simulink model "PMfinal"  (R2018a)
settings: Solver=VariableStepDiscrete  StartTime=0.0  StopTime=10.0  RelTol=1e-3
libraries: powerlib x16, simulink x3, powerlib_meascontrol x1
settings Model: Creator=enes_  LastModifiedBy=enes_

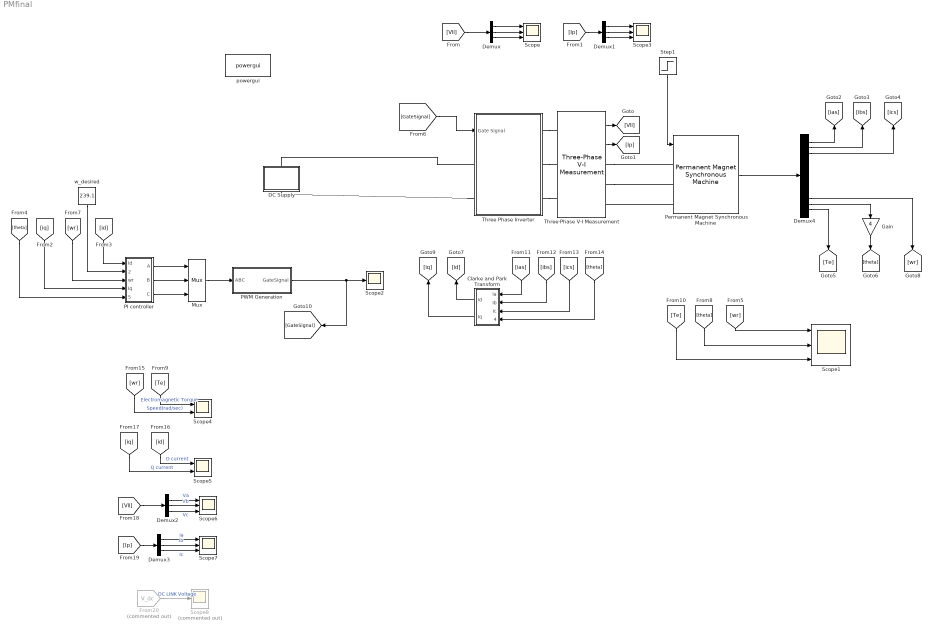
== system PMfinal ==
  Clarke and Park Transform : Subsystem
  DC Supply : Subsystem
  Demux{,1..3} (4 alike) : Demux  Outputs=3
  Demux4 : Demux  Outputs=13
  From20 : From  Commented=on  GotoTag=V_dc  TagVisibility=global
  Gain : Gain  Gain=4
  Mux : Mux  Inputs=3
  PI controller : Subsystem
  PWM Generation : Subsystem
  Permanent Magnet Synchronous Machine : powerlib/Machines/Permanent Magnet Synchronous Machine  NbPhases=3  FluxDistribution=Sinusoidal  RotorType=Round  MechanicalLoad=Torque Tm  PresetModel=No  ShowDetailedParameters=on  MeasurementBus=off  Resistance=50e-3  Inductance=8.5e-3  dqInductances=[500e-6,500e-6]  La=500e-6  MachineConstant=Flux linkage established by magnets (V.s)  Flux=0.2  VoltageCst=145.1039  TorqueCst=1.2  Flat=120  Mechanical=[10 0 4 0]  PolePairs=4  InitialConditions=[266,0, 0,0]  InitialConditions5ph=[266 0 0 0 0 0]  TsPowergui=0  TsBlock=-1  RefAngle=Aligned with phase A axis (original Park)
  Scope{,1,3,6..7} (5 alike) : Scope  NumInputPorts=3
  Scope2 : Scope
  Scope4 : Scope  NumInputPorts=2
  Scope5 : Scope  NumInputPorts=2
  Scope8 : Scope  Commented=on
  Step1 : Step  Time=.1  After=60  SampleTime=1e-6
  Three Phase Inverter : Subsystem  RequirementInfo="{}  %GIDa_97822f1e_2a67_44f0_8b0b_8fc93499e893"
  Three-Phase V-I Measurement : powerlib/Measurements/Three-Phase V-I Measurement  VoltageMeasurement=phase-to-phase  SetLabelV=off  LabelV=Vabc  Vpu=off  VpuLL=off  CurrentMeasurement=yes  SetLabelI=off  LabelI=Iabc  Ipu=off  Pbase=100e6  Vbase=500e3  OutputType=Complex  PhasorSimulation=off  PSBequivalent=0
      settings: SourceProductName=Simscape Electrical
  powergui : powerlib/powergui  Priority=1  SimulationMode=Discrete  SampleTime=1e-6  frequency=60  Iterations=50  frequencyindice=0  Pbase=100e6  ErrMax=1e-4  UnitsV=kV  UnitsW=MW  buscounter=0  FunctionMessages=off  echomessages=off  EnableUseOfTLC=off  CurrentSourceSwitches=off  DisableSnubberDevices=off  DisableRonSwitches=off  DisableVfSwitches=off  DisplayEquations=off  SolverType=Tustin/Backward Euler (TBE)  Interpol=off  ExternalGateDelay=off  methode=off  Ts=100  x0status=blocks  SPID=on  SwTol=0  HookPort=off  RestoreLinks=warning  ResistiveCurrentMeasurement=off  Frange=[0:2:500]  Ylog=off  Xlog=on  ShowGrid=off  save=off  variable=ZData  structure=0  ZoomFFT=off  StartTime=0.0  cycles=1  DisplayStyle=1  fundamental=60  FreqAxis=off  MaxFrequency=1000  frequencyindicesteady=1  RmsSteady=1  display=off
  w_desired : Constant  Value=239.1
  wires:
  Step1/1 -> Permanent Magnet Synchronous Machine/1
  Three-Phase V-I Measurement/1 -> [Vll]
  [Vll] -> Demux/1
  Demux/1 -> Scope/1
  Demux/2 -> Scope/2
  Demux/3 -> Scope/3
  Three-Phase V-I Measurement/2 -> [Ip]
  [Ip] -> Demux1/1
  Demux1/1 -> Scope3/1
  Demux1/2 -> Scope3/2
  Demux1/3 -> Scope3/3
  Permanent Magnet Synchronous Machine/1 -> Demux4/1
  Demux4/1 -> [ias]
  Demux4/2 -> [ibs]
  Demux4/3 -> [ics]
  Demux4/13 -> [Te]
  Demux4/12 -> Gain/1
  Demux4/11 -> [wr]
  Gain/1 -> [theta]
  [wr] -> Scope1/1
  [theta] -> Scope1/2
  [Te] -> Scope1/3
  PWM Generation/1("GateSignal ") -> Scope2/1, [GateSignal]
  Mux/1 -> PWM Generation/1(ABC)
  [GateSignal] -> Three Phase Inverter/1(Gate Signal)
  [ias] -> Clarke and Park Transform/1(Ia)
  [ibs] -> Clarke and Park Transform/2(Ib)
  [ics] -> Clarke and Park Transform/3(Ic)
  [theta] -> Clarke and Park Transform/4(Theta)
  Clarke and Park Transform/1(Id) -> [id]
  Clarke and Park Transform/2(Iq) -> [iq]
  [id] -> PI controller/1(Id)
  w_desired/1 -> PI controller/2(w_ref)
  [wr] -> PI controller/3(wr)
  [iq] -> PI controller/4(Iq)
  [theta] -> PI controller/5(Theta)
  PI controller/1(A) -> Mux/1
  PI controller/2(B) -> Mux/2
  PI controller/3(C) -> Mux/3
  [Te] -> Scope4/1  "Electromagnetic Torque"
  [wr] -> Scope4/2  "Speed(rad/sec)"
  [id] -> Scope5/1  "D current"
  [iq] -> Scope5/2  "Q current"
  Demux3/2 -> Scope7/2  "Ib"
  Demux2/2 -> Scope6/2  "Vb"
  [Vll] -> Demux2/1
  Demux3/1 -> Scope7/1  "Ia"
  Demux2/3 -> Scope6/3  "Vc"
  [Ip] -> Demux3/1
  Demux3/3 -> Scope7/3  "Ic"
  Demux2/1 -> Scope6/1  "Va"
  From20/1 -> Scope8/1  "DC LINK Voltage"
  connections:
  Three Phase Inverter/LConn2 -- DC Supply/LConn1
  DC Supply/RConn1 -- Three Phase Inverter/LConn1
  Three-Phase V-I Measurement/RConn1 -- Permanent Magnet Synchronous Machine/LConn1
  Three-Phase V-I Measurement/RConn2 -- Permanent Magnet Synchronous Machine/LConn2
  Permanent Magnet Synchronous Machine/LConn3 -- Three-Phase V-I Measurement/RConn3
  Three Phase Inverter/RConn1 -- Three-Phase V-I Measurement/LConn1
  Three Phase Inverter/RConn2 -- Three-Phase V-I Measurement/LConn2
  Three Phase Inverter/RConn3 -- Three-Phase V-I Measurement/LConn3

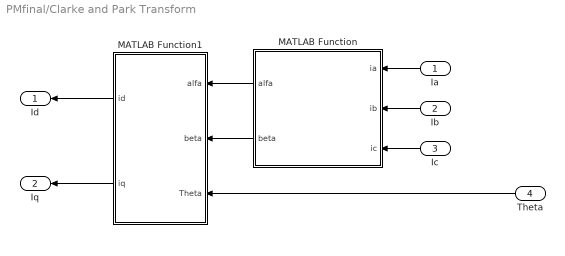
== system PMfinal/Clarke and Park Transform ==
  Ia : Inport
  Ib : Inport  Port=2
  Ic : Inport  Port=3
  Theta : Inport  Port=4
  MATLAB Function : MATLAB Function  TreatAsAtomicUnit=on
  MATLAB Function1 : MATLAB Function  TreatAsAtomicUnit=on
  Id : Outport
  Iq : Outport  Port=2
  wires:
  Ib/1 -> MATLAB Function/2(ib)
  MATLAB Function/2(beta) -> MATLAB Function1/2(beta)
  Ia/1 -> MATLAB Function/1(ia)
  MATLAB Function/1(alfa) -> MATLAB Function1/1(alfa)
  Theta/1 -> MATLAB Function1/3(Theta)
  MATLAB Function1/2(iq) -> Iq/1
  Ic/1 -> MATLAB Function/3(ic)
  MATLAB Function1/1(id) -> Id/1

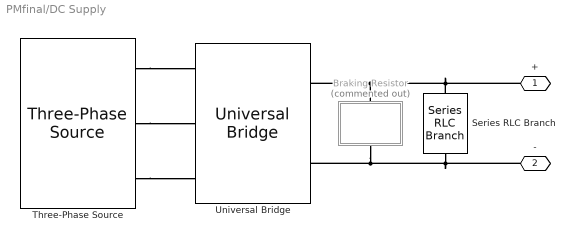
== system PMfinal/DC Supply ==
  "Braking Resistor " : Subsystem  Commented=on
  Series RLC Branch : powerlib/Elements/Series RLC Branch  LConnTagsString=__new0  RConnTagsString=__new0  BranchType=C  Resistance=1  Inductance=1e-3  SetiL0=off  InitialCurrent=0  Capacitance=330e-3  Setx0=off  InitialVoltage=0  Measurements=None
      settings: SourceProductName=Simscape Electrical
  "Three-Phase Source " : powerlib/Electrical Sources/Three-Phase Source  InternalConnection=Yg  VoltagePhases=off  Voltage=400  PhaseAngle=0  Voltage_phases=[25e3 25e3 25e3]/sqrt(3)  PhaseAngles_phases=[0 -120 +120]  Frequency=50  NonIdealSource=off  SpecifyImpedance=off  Resistance=0  Inductance=0  ShortCircuitLevel=100e6  BaseVoltage=25e3  XRratio=7  BusType=swing  Pref=10e3  Qref=0  Prefabc=[10e3, 10e3, 10e3]  Qrefabc=[0, 0, 0]  Qmin=-inf  Qmax=inf
      settings: SourceProductName=Simscape Electrical
  "Universal Bridge " : powerlib/Power Electronics/Universal Bridge  Arms=3  SnubberResistance=1e5  SnubberCapacitance=inf  Device=Diodes  Ron=1e-3  Lon=0  ForwardVoltages="[  0  0  ]"  ForwardVoltage=0  GTOparameters=[ 10e-6 , 20e-6 ]  IGBTparameters=[ 1e-6 , 2e-6 ]  Measurements=All voltages and currents  Measurements_2=None  converterType=Rectifier
      settings: SourceProductName=Simscape Electrical
  + : PMIOPort  Side=Right
  - : PMIOPort  Port=2  Side=Left
  connections:
  "Three-Phase Source "/RConn3 -- "Universal Bridge "/LConn3
  Series RLC Branch/RConn1 -- -/RConn1 -- "Braking Resistor "/RConn1 -- "Universal Bridge "/RConn2
  Series RLC Branch/LConn1 -- "Braking Resistor "/LConn1 -- "Universal Bridge "/RConn1 -- +/RConn1
  "Three-Phase Source "/RConn1 -- "Universal Bridge "/LConn1
  "Three-Phase Source "/RConn2 -- "Universal Bridge "/LConn2

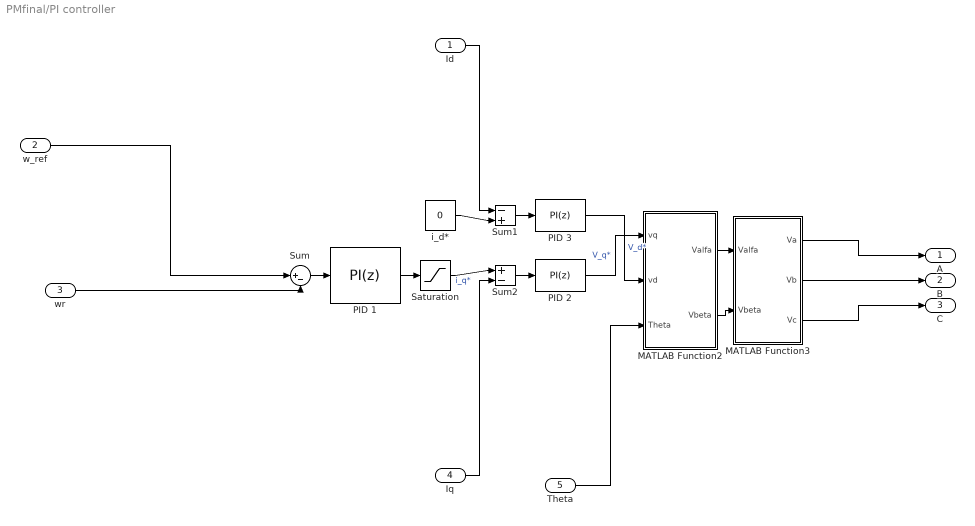
== system PMfinal/PI controller ==
  Id : Inport
  w_ref : Inport  Port=2
  wr : Inport  Port=3
  Iq : Inport  Port=4
  Theta : Inport  Port=5
  MATLAB Function2 : MATLAB Function  TreatAsAtomicUnit=on
  MATLAB Function3 : MATLAB Function  TreatAsAtomicUnit=on
  PID 1 : simulink/Continuous/PID Controller  Controller=PI  TimeDomain=Discrete-time  SampleTime=-1  IntegratorMethod=Forward Euler  FilterMethod=Forward Euler  Form=Parallel  UseFilter=on  ControllerParametersSource=internal  P=990  I=6  D=0  N=100  InitialConditionSource=internal  InitialConditionForIntegrator=0  InitialConditionForFilter=0  ExternalReset=none  LimitOutput=off  UpperSaturationLimit=inf  LowerSaturationLimit=-inf  LinearizeAsGain=on  AntiWindupMode=none  Kb=1  TrackingMode=off  Kt=1  PParamMin=[]  PParamMax=[]  IParamMin=[]  IParamMax=[]  DParamMin=[]  DParamMax=[]  NParamMin=[]  NParamMax=[]  KbParamMin=[]  KbParamMax=[]  KtParamMin=[]  KtParamMax=[]  POutMin=[]  POutMax=[]  IOutMin=[]  IOutMax=[]  DOutMin=[]  DOutMax=[]  NOutMin=[]  NOutMax=[]  KbOutMin=[]  KbOutMax=[]  KtOutMin=[]  KtOutMax=[]  IntegratorOutMin=[]  IntegratorOutMax=[]  FilterOutMin=[]  FilterOutMax=[]  SumOutMin=[]  SumOutMax=[]  SumI1OutMin=[]  SumI1OutMax=[]  SumI2OutMin=[]  SumI2OutMax=[]  SumI3OutMin=[]  SumI3OutMax=[]  SumDOutMin=[]  SumDOutMax=[]  SaturationOutMin=[]  SaturationOutMax=[]  IntegratorContinuousStateAttributes=''  IntegratorStateMustResolveToSignalObject=off  IntegratorRTWStateStorageClass=Auto  FilterContinuousStateAttributes=''  FilterStateMustResolveToSignalObject=off  FilterRTWStateStorageClass=Auto  DifferentiatorICPrevScaledInput=0  DifferentiatorOutMin=[]  DifferentiatorOutMax=[]  FilterDiffOutCoefMin=[]  FilterDiffOutCoefMax=[]  SumDenOutMin=[]  SumDenOutMax=[]  SumNumOutMin=[]  SumNumOutMax=[]  ReciprocalOutMin=[]  ReciprocalOutMax=[]  DivideOutMin=[]  DivideOutMax=[]  TunerSelectOption=Transfer Function Based (PID Tuner App)
  PID 2 : simulink/Continuous/PID Controller  Controller=PI  TimeDomain=Discrete-time  SampleTime=-1  IntegratorMethod=Forward Euler  FilterMethod=Forward Euler  Form=Parallel  UseFilter=on  ControllerParametersSource=internal  P=1  I=990  D=0.1  N=100  InitialConditionSource=internal  InitialConditionForIntegrator=0  InitialConditionForFilter=0  ExternalReset=none  LimitOutput=off  UpperSaturationLimit=inf  LowerSaturationLimit=-inf  LinearizeAsGain=on  AntiWindupMode=none  Kb=1  TrackingMode=off  Kt=1  PParamMin=[]  PParamMax=[]  IParamMin=[]  IParamMax=[]  DParamMin=[]  DParamMax=[]  NParamMin=[]  NParamMax=[]  KbParamMin=[]  KbParamMax=[]  KtParamMin=[]  KtParamMax=[]  POutMin=[]  POutMax=[]  IOutMin=[]  IOutMax=[]  DOutMin=[]  DOutMax=[]  NOutMin=[]  NOutMax=[]  KbOutMin=[]  KbOutMax=[]  KtOutMin=[]  KtOutMax=[]  IntegratorOutMin=[]  IntegratorOutMax=[]  FilterOutMin=[]  FilterOutMax=[]  SumOutMin=[]  SumOutMax=[]  SumI1OutMin=[]  SumI1OutMax=[]  SumI2OutMin=[]  SumI2OutMax=[]  SumI3OutMin=[]  SumI3OutMax=[]  SumDOutMin=[]  SumDOutMax=[]  SaturationOutMin=[]  SaturationOutMax=[]  IntegratorContinuousStateAttributes=''  IntegratorStateMustResolveToSignalObject=off  IntegratorRTWStateStorageClass=Auto  FilterContinuousStateAttributes=''  FilterStateMustResolveToSignalObject=off  FilterRTWStateStorageClass=Auto  DifferentiatorICPrevScaledInput=0  DifferentiatorOutMin=[]  DifferentiatorOutMax=[]  FilterDiffOutCoefMin=[]  FilterDiffOutCoefMax=[]  SumDenOutMin=[]  SumDenOutMax=[]  SumNumOutMin=[]  SumNumOutMax=[]  ReciprocalOutMin=[]  ReciprocalOutMax=[]  DivideOutMin=[]  DivideOutMax=[]  TunerSelectOption=Transfer Function Based (PID Tuner App)
  PID 3 : simulink/Continuous/PID Controller  Controller=PI  TimeDomain=Discrete-time  SampleTime=-1  IntegratorMethod=Forward Euler  FilterMethod=Forward Euler  Form=Parallel  UseFilter=on  ControllerParametersSource=internal  P=1  I=990  D=0.1  N=100  InitialConditionSource=internal  InitialConditionForIntegrator=0  InitialConditionForFilter=0  ExternalReset=none  LimitOutput=off  UpperSaturationLimit=inf  LowerSaturationLimit=-inf  LinearizeAsGain=on  AntiWindupMode=none  Kb=1  TrackingMode=off  Kt=1  PParamMin=[]  PParamMax=[]  IParamMin=[]  IParamMax=[]  DParamMin=[]  DParamMax=[]  NParamMin=[]  NParamMax=[]  KbParamMin=[]  KbParamMax=[]  KtParamMin=[]  KtParamMax=[]  POutMin=[]  POutMax=[]  IOutMin=[]  IOutMax=[]  DOutMin=[]  DOutMax=[]  NOutMin=[]  NOutMax=[]  KbOutMin=[]  KbOutMax=[]  KtOutMin=[]  KtOutMax=[]  IntegratorOutMin=[]  IntegratorOutMax=[]  FilterOutMin=[]  FilterOutMax=[]  SumOutMin=[]  SumOutMax=[]  SumI1OutMin=[]  SumI1OutMax=[]  SumI2OutMin=[]  SumI2OutMax=[]  SumI3OutMin=[]  SumI3OutMax=[]  SumDOutMin=[]  SumDOutMax=[]  SaturationOutMin=[]  SaturationOutMax=[]  IntegratorContinuousStateAttributes=''  IntegratorStateMustResolveToSignalObject=off  IntegratorRTWStateStorageClass=Auto  FilterContinuousStateAttributes=''  FilterStateMustResolveToSignalObject=off  FilterRTWStateStorageClass=Auto  DifferentiatorICPrevScaledInput=0  DifferentiatorOutMin=[]  DifferentiatorOutMax=[]  FilterDiffOutCoefMin=[]  FilterDiffOutCoefMax=[]  SumDenOutMin=[]  SumDenOutMax=[]  SumNumOutMin=[]  SumNumOutMax=[]  ReciprocalOutMin=[]  ReciprocalOutMax=[]  DivideOutMin=[]  DivideOutMax=[]  TunerSelectOption=Transfer Function Based (PID Tuner App)
  Saturation : Saturate  UpperLimit=250  LowerLimit=-250
  Sum : Sum  Inputs=|+-
  Sum1 : Sum  Inputs=-+|
  Sum2 : Sum  Inputs=|+-
  i_d* : Constant  Value=0
  A : Outport
  B : Outport  Port=2
  C : Outport  Port=3
  wires:
  MATLAB Function2/1(Valfa) -> MATLAB Function3/1(Valfa)
  PID 2/1 -> MATLAB Function2/1(vq)  "V_q*"
  i_d*/1 -> Sum1/2
  Id/1 -> Sum1/1
  Sum1/1 -> PID 3/1
  Saturation/1 -> Sum2/1  "i_q*"
  Sum2/1 -> PID 2/1
  PID 1/1 -> Saturation/1
  Sum/1 -> PID 1/1
  MATLAB Function3/1(Va) -> A/1
  PID 3/1 -> MATLAB Function2/2(vd)  "V_d*"
  MATLAB Function2/2(Vbeta) -> MATLAB Function3/2(Vbeta)
  Theta/1 -> MATLAB Function2/3(Theta)
  Iq/1 -> Sum2/2
  MATLAB Function3/3(Vc) -> C/1
  wr/1 -> Sum/2
  MATLAB Function3/2(Vb) -> B/1
  w_ref/1 -> Sum/1

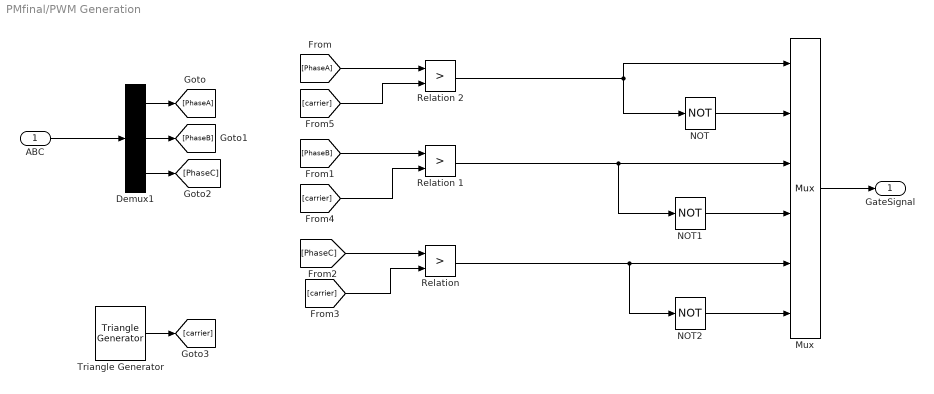
== system PMfinal/PWM Generation ==
  ABC : Inport
  Demux1 : Demux  Outputs=3
  Mux : Mux  Inputs=6
  NOT : Logic  Operator=NOT  IconShape=distinctive  AllPortsSameDT=off  OutDataTypeStr=boolean
  NOT1 : Logic  Operator=NOT  IconShape=distinctive  AllPortsSameDT=off  OutDataTypeStr=boolean
  NOT2 : Logic  Operator=NOT  IconShape=distinctive  AllPortsSameDT=off  OutDataTypeStr=boolean
  "Relation " : RelationalOperator  Operator=>  OutDataTypeStr=boolean  RndMeth=Simplest
  Relation 1 : RelationalOperator  Operator=>  OutDataTypeStr=boolean  RndMeth=Simplest
  Relation 2 : RelationalOperator  Operator=>  OutDataTypeStr=boolean  RndMeth=Simplest
  Triangle Generator : powerlib_meascontrol/Pulse & Signal Generators/Triangle Generator  Freq=1e4  Phase=0  Ts=0
  "GateSignal " : Outport
  wires:
  ABC/1 -> Demux1/1
  [PhaseA] -> Relation 2/1
  Demux1/1 -> [PhaseA]
  [PhaseB] -> Relation 1/1
  Demux1/2 -> [PhaseB]
  Demux1/3 -> [PhaseC]
  [PhaseC] -> "Relation "/1
  Triangle Generator/1 -> [carrier]
  [carrier] -> "Relation "/2
  [carrier] -> Relation 1/2
  [carrier] -> Relation 2/2
  Mux/1 -> "GateSignal "/1
  NOT/1 -> Mux/2
  NOT1/1 -> Mux/4
  Relation 2/1 -> NOT/1, Mux/1
  Relation 1/1 -> Mux/3, NOT1/1
  "Relation "/1 -> Mux/5, NOT2/1
  NOT2/1 -> Mux/6

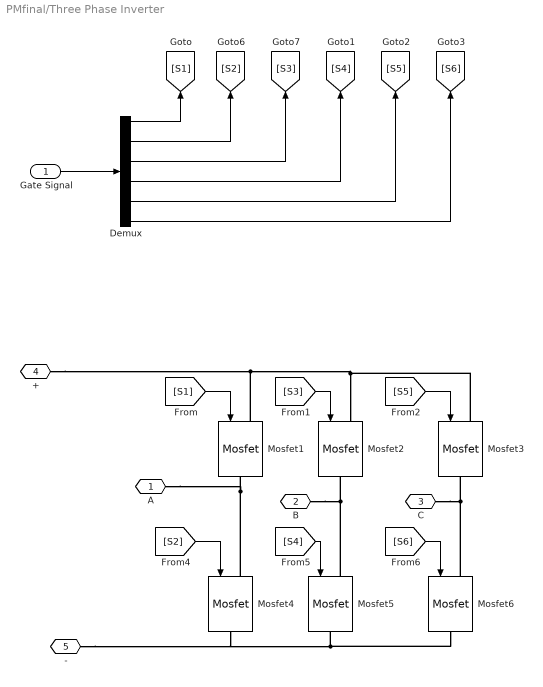
== system PMfinal/Three Phase Inverter ==
  Gate Signal : Inport
  Demux : Demux  Outputs=6
  Mosfet{1..6} (6 alike) : powerlib/Power Electronics/Mosfet  Ron=0.1  Lon=0  Rd=0.01  Vfd=0.7  IC=0  Rs=1e5  Cs=inf  Measurements=off
  A : PMIOPort  Side=Right
  B : PMIOPort  Port=2  Side=Right
  C : PMIOPort  Port=3  Side=Right
  + : PMIOPort  Port=4  Side=Left
  - : PMIOPort  Port=5  Side=Left
  wires:
  Gate Signal/1 -> Demux/1
  Demux/1 -> [S1]
  Demux/2 -> [S2]
  Demux/3 -> [S3]
  Demux/4 -> [S4]
  Demux/5 -> [S5]
  Demux/6 -> [S6]
  [S1] -> Mosfet1/1
  [S3] -> Mosfet2/1
  [S5] -> Mosfet3/1
  [S2] -> Mosfet4/1
  [S4] -> Mosfet5/1
  [S6] -> Mosfet6/1
  connections:
  Mosfet6/LConn1 -- C/RConn1 -- Mosfet3/RConn1
  Mosfet5/LConn1 -- B/RConn1 -- Mosfet2/RConn1
  Mosfet4/LConn1 -- A/RConn1 -- Mosfet1/RConn1
  Mosfet1/LConn1 -- Mosfet3/LConn1 -- Mosfet2/LConn1 -- +/RConn1
  Mosfet6/RConn1 -- -/RConn1 -- Mosfet4/RConn1 -- Mosfet5/RConn1

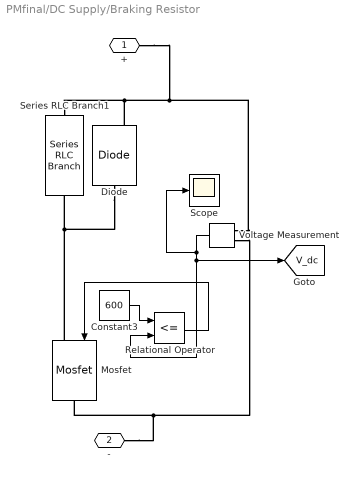
== system PMfinal/DC Supply/Braking Resistor  ==
  Constant3 : Constant  Value=600
  Diode : powerlib/Power Electronics/Diode  Ron=0.001  Lon=0  Vf=0.8  IC=0  UseSnubber=0  Rs=500  Cs=250e-9  Measurements=on
  Mosfet : powerlib/Power Electronics/Mosfet  Ron=0.1  Lon=0  Rd=0.01  Vfd=0  IC=0  Rs=1e5  Cs=inf  Measurements=off
      settings: SourceProductName=Simscape Electrical
  Relational Operator : RelationalOperator  Operator=<=  OutDataTypeStr=boolean  RndMeth=Simplest
  Scope : Scope
  Series RLC Branch1 : powerlib/Elements/Series RLC Branch  LConnTagsString=__new0  RConnTagsString=__new0  BranchType=R  Resistance=5  Inductance=1e-3  SetiL0=off  InitialCurrent=0  Capacitance=1e-6  Setx0=off  InitialVoltage=0  Measurements=None
  Voltage Measurement : powerlib/Measurements/Voltage Measurement  PhasorSimulation=off  OutputType=Complex  PSBequivalent=0
      settings: SourceProductName=Simscape Electrical
  + : PMIOPort  Side=Left
  - : PMIOPort  Port=2  Side=Right
  tag scope: V_dc=global
  wires:
  Voltage Measurement/1 -> Scope/1, [V_dc], Relational Operator/2
  Relational Operator/1 -> Mosfet/1
  Constant3/1 -> Relational Operator/1
  connections:
  Diode/LConn1 -- Mosfet/LConn1 -- Series RLC Branch1/RConn1
  Voltage Measurement/LConn2 -- -/RConn1 -- Mosfet/RConn1
  Voltage Measurement/LConn1 -- +/RConn1 -- Diode/RConn1 -- Series RLC Branch1/LConn1

== matlab function PMfinal/Clarke and Park Transform/MATLAB Function1 ==
  data: alfa input; id output; beta input; Theta input; iq output
function [id,iq]= dqTransform(alfa,beta,Theta)
id= cos(Theta)*alfa+ sin(Theta)*beta;
iq=-sin(Theta)*alfa+ cos(Theta)*beta;

== matlab function PMfinal/Clarke and Park Transform/MATLAB Function ==
  data: ia input; alfa output; ib input; ic input; beta output
function [alfa,beta]= alfaBetaConversion(ia,ib,ic)
alfa= (2/3)* (ia -ib/2 - ic/2);
beta =(2/3)*( sqrt(3)*ib/2 - sqrt(3)*ic/2);

== matlab function PMfinal/PI controller/MATLAB Function2 ==
  data: vq input; Valfa output; vd input; Theta input; Vbeta output
function [Valfa,Vbeta]= fcn(vq,vd,Theta)

Valfa=cos(Theta)*vd -sin(Theta)*vq;
Vbeta=sin(Theta)*vd+ cos(Theta)*vq;

== matlab function PMfinal/PI controller/MATLAB Function3 ==
  data: Valfa input; Va output; Vbeta input; Vb output; Vc output
function [Va,Vb,Vc]= fcn(Valfa,Vbeta)
Va=Valfa;
Vb=( -Valfa+ sqrt(3)*Vbeta)/2;
Vc=( -Valfa- sqrt(3)*Vbeta)/2;
